simulink model "IndustrialMicrogrid"  (R2025a)
settings: Solver=FixedStepAuto  StartTime=0.0  StopTime=8  FixedStep=Ts  RelTol=1e-3
PostLoadFcn:
  | IndustrialMicrogridInputData
  | GfmGridFormingConverterInputParameters
model workspace (MAT data in the model file):
  caseNum = 2
undefined symbols (not defined in the file): base, BESS, DiscIntNeverNeededParam, grid, Grid, gridInverter, machine, microgrid, PV, PVInverter, PVTransformer, scrFactorRg, scrFactorXg, transformer, Transition_and_Dispatch_ControlModeType, Ts
libraries: ee_lib x126, fl_lib x91, eeGeneralControl x73, nesl_utility x50, nesl_utility_internal x46, simulink x30, eeTransforms x11, eeSinusoidalMeasurementV2 x5, eeTotalHarmonicDistorsion x4, slpidlib x3, simulink_extras x2, eePowerMeasurement x2
(part 7 of 12)

== system IndustrialMicrogrid/MG2 Primary Substation/PCC Measurements and PCC Breaker/Circuit Breaker ==
  BRK : Inport
  Data Type Conversion : DataTypeConversion  OutDataTypeStr=double  SaturateOnIntegerOverflow=off  RndMeth=Floor
  Open Resistance : Gain  Gain=5e6
  Phase Splitter : ee_lib/Connectors & References/Phase Splitter
  Phase Splitter1 : ee_lib/Connectors & References/Phase Splitter
  Simulink-PS Converter : nesl_utility/Simulink-PS Converter  PhysicalDomain=network_engine_domain  SubClassName=ps_input  LeftPortType=input  RightPortType=output  PseudoPeriodic=off  Frequencies=[]  NoiseDistribution=none  NoiseParameters=[]  Unit=1  AffineConversion=off  FilteringAndDerivatives=provide  SimscapeFilterOrder=1  InputFilterTimeConstant=0.001  UdotUserProvided=0
  Variable Resistor : fl_lib/Electrical/Electrical Elements/Variable Resistor  Rmin=1e-3 Ohm  thermalEnable=false  thermal_mass=1 J/K  i_specify=off  i_priority=None  i=0 A  i_nominal_specify=off  i_nominal_value=1  i_nominal_unit=A  v_specify=off  v_priority=None  v=0 V  v_nominal_specify=off  v_nominal_value=1  v_nominal_unit=V  T_specify=off  T_priority=None  T=300 K  T_nominal_specify=off  T_nominal_value=1  T_nominal_unit=K
  Variable Resistor1 : fl_lib/Electrical/Electrical Elements/Variable Resistor  Rmin=1e-3 Ohm  thermalEnable=false  thermal_mass=1 J/K  i_specify=off  i_priority=None  i=0 A  i_nominal_specify=off  i_nominal_value=1  i_nominal_unit=A  v_specify=off  v_priority=None  v=0 V  v_nominal_specify=off  v_nominal_value=1  v_nominal_unit=V  T_specify=off  T_priority=None  T=300 K  T_nominal_specify=off  T_nominal_value=1  T_nominal_unit=K
  Variable Resistor2 : fl_lib/Electrical/Electrical Elements/Variable Resistor  Rmin=1e-3 Ohm  thermalEnable=false  thermal_mass=1 J/K  i_specify=off  i_priority=None  i=0 A  i_nominal_specify=off  i_nominal_value=1  i_nominal_unit=A  v_specify=off  v_priority=None  v=0 V  v_nominal_specify=off  v_nominal_value=1  v_nominal_unit=V  T_specify=off  T_priority=None  T=300 K  T_nominal_specify=off  T_nominal_value=1  T_nominal_unit=K
  In : PMIOPort  Side=Left
  ~ : PMIOPort  Port=2  Side=Right
  wires:
  Data Type Conversion/1 -> Open Resistance/1
  BRK/1 -> Data Type Conversion/1
  Open Resistance/1 -> Simulink-PS Converter/1
  connections:
  Phase Splitter1/RConn2 -- Variable Resistor1/RConn1
  Variable Resistor1/LConn2 -- Phase Splitter/RConn2
  Phase Splitter1/RConn3 -- Variable Resistor2/RConn1
  Phase Splitter/RConn1 -- Variable Resistor/LConn2
  Variable Resistor2/LConn2 -- Phase Splitter/RConn3
  Phase Splitter1/RConn1 -- Variable Resistor/RConn1
  Phase Splitter1/LConn1 -- ~/RConn1
  Variable Resistor/LConn1 -- Simulink-PS Converter/RConn1 -- Variable Resistor2/LConn1 -- Variable Resistor1/LConn1
  Phase Splitter/LConn1 -- In/RConn1

== system IndustrialMicrogrid/MG2 Primary Substation/PCC Measurements and PCC Breaker/Grid Current Measurement ==
  Current and Voltage Sensor (Three-Phase)1 : ee_lib/Sensors & Transducers/Current and Voltage Sensor (Three-Phase)  vMeasurementType=ee.enum.vmeasurement.ll  outputUnit=ee.enum.unit.pu  SRated=2.5e6 A*V  VRated=microgrid.voltage V  I_specify=off  I_priority=None  I=[0, 0, 0] A  I_nominal_specify=off  I_nominal_value=1  I_nominal_unit=A  V_specify=off  V_priority=None  V=[0, 0, 0] V  V_nominal_specify=off  V_nominal_value=1  V_nominal_unit=V
      settings: InternalSimscapePortConfiguration="{\"Bottom\":[],\"Left\":[{\"id\":\"N1\",\"label\":\"~1\",\"type\":\"foundation.electrical.three_phase\"}],\"Right\":[{\"id\":\"V_output\",\"label\":\"V\",\"type\":\"output\"},{\"id\":\"I_output\",\"label\":\"I\",\"type\":\"output\"},{\"id\":\"N2\",\"label\":\"~2\",\"type\":\"foundation.electrical.three_phase\"}],\"Top\":[]}"
  PS-Simulink Converter2 : nesl_utility_internal/PS-Simulink Converter  PhysicalDomain=network_engine_domain  SubClassName=ps_output  LeftPortType=input  RightPortType=output  PseudoPeriodic=off  Frequencies=[]  VectorFormat=1-D array  Unit=V  AffineConversion=off
  PS-Simulink Converter3 : nesl_utility_internal/PS-Simulink Converter  PhysicalDomain=network_engine_domain  SubClassName=ps_output  LeftPortType=input  RightPortType=output  PseudoPeriodic=off  Frequencies=[]  VectorFormat=1-D array  Unit=A  AffineConversion=off
  Terminator : Terminator
  ~ : PMIOPort  Side=Left
  "~ " : PMIOPort  Port=2  Side=Right
  Out Bus Element : Outport  PortName=Grid  Element=voltage
  wires:
  PS-Simulink Converter3/1 -> Terminator/1
  PS-Simulink Converter2/1 -> Out Bus Element/1
  connections:
  Current and Voltage Sensor (Three-Phase)1/RConn3 -- "~ "/RConn1
  Current and Voltage Sensor (Three-Phase)1/RConn2 -- PS-Simulink Converter3/LConn1
  ~/RConn1 -- Current and Voltage Sensor (Three-Phase)1/LConn1
  Current and Voltage Sensor (Three-Phase)1/RConn1 -- PS-Simulink Converter2/LConn1

== system IndustrialMicrogrid/MG2 Primary Substation/PCC Measurements and PCC Breaker/Grid Power Measurement ==
  Current and Voltage Sensor (Three-Phase) : ee_lib/Sensors & Transducers/Current and Voltage Sensor (Three-Phase)  vMeasurementType=ee.enum.vmeasurement.ll  outputUnit=ee.enum.unit.pu  SRated=2.5e6 A*V  VRated=microgrid.voltage V  I_specify=off  I_priority=None  I=[0, 0, 0] A  I_nominal_specify=off  I_nominal_value=1  I_nominal_unit=A  V_specify=off  V_priority=None  V=[0, 0, 0] V  V_nominal_specify=off  V_nominal_value=1  V_nominal_unit=V
      settings: InternalSimscapePortConfiguration="{\"Bottom\":[],\"Left\":[{\"id\":\"N1\",\"label\":\"~1\",\"type\":\"foundation.electrical.three_phase\"}],\"Right\":[{\"id\":\"V_output\",\"label\":\"V\",\"type\":\"output\"},{\"id\":\"I_output\",\"label\":\"I\",\"type\":\"output\"},{\"id\":\"N2\",\"label\":\"~2\",\"type\":\"foundation.electrical.three_phase\"}],\"Top\":[]}"
  Low-Pass Filter (Discrete or Continuous) : eeGeneralControl/Low-Pass Filter (Discrete or Continuous)  K=1  T=0.1  B=inf  A=-inf  init_option=Inherited from block input  x0=0  Ts=Ts
  Low-Pass Filter (Discrete or Continuous)1 : eeGeneralControl/Low-Pass Filter (Discrete or Continuous)  K=1  T=0.1  B=inf  A=-inf  init_option=Inherited from block input  x0=0  Ts=Ts
  PS-Simulink Converter : nesl_utility_internal/PS-Simulink Converter  PhysicalDomain=network_engine_domain  SubClassName=ps_output  LeftPortType=input  RightPortType=output  PseudoPeriodic=off  Frequencies=[]  VectorFormat=1-D array  Unit=inherit  AffineConversion=off
  PS-Simulink Converter1 : nesl_utility_internal/PS-Simulink Converter  PhysicalDomain=network_engine_domain  SubClassName=ps_output  LeftPortType=input  RightPortType=output  PseudoPeriodic=off  Frequencies=[]  VectorFormat=1-D array  Unit=inherit  AffineConversion=off
  PS-Simulink Converter8 : nesl_utility_internal/PS-Simulink Converter  PhysicalDomain=network_engine_domain  SubClassName=ps_output  LeftPortType=input  RightPortType=output  PseudoPeriodic=off  Frequencies=[]  VectorFormat=1-D array  Unit=MW  AffineConversion=off
  PS-Simulink Converter9 : nesl_utility_internal/PS-Simulink Converter  PhysicalDomain=network_engine_domain  SubClassName=ps_output  LeftPortType=input  RightPortType=output  PseudoPeriodic=off  Frequencies=[]  VectorFormat=1-D array  Unit=MV*A  AffineConversion=off
  Power Sensor (Three-Phase)2 : ee_lib/Sensors & Transducers/Power Sensor (Three-Phase)  load_type=ee.enum.passive.type_balanced.balanced  f0=60 Hz  config=ee.enum.with_neutral.no  rho=1
      settings: InternalSimscapePortConfiguration="{\"Bottom\":[],\"Left\":[{\"id\":\"N1\",\"label\":\"~1\",\"type\":\"foundation.electrical.three_phase\"}],\"Right\":[{\"id\":\"N2\",\"label\":\"~2\",\"type\":\"foundation.electrical.three_phase\"}],\"Top\":[{\"id\":\"Pm\",\"label\":\"P\",\"type\":\"output\"},{\"id\":\"Qm\",\"label\":\"Q\",\"type\":\"output\"}]}"
  ~ : PMIOPort  Side=Left
  "~ " : PMIOPort  Port=2  Side=Right
  Out Bus Element : Outport  PortName=PCC  Element=voltage
  Out Bus Element1 : Outport  PortName=PCC  Element=current
  Out Bus Element2 : Outport  PortName=PCC  Element=activePower
  Out Bus Element3 : Outport  PortName=PCC  Element=reactivePower
  wires:
  Low-Pass Filter (Discrete or Continuous)1/1 -> Out Bus Element3/1
  Low-Pass Filter (Discrete or Continuous)/1 -> Out Bus Element2/1
  PS-Simulink Converter1/1 -> Out Bus Element1/1
  PS-Simulink Converter/1 -> Out Bus Element/1
  PS-Simulink Converter9/1 -> Low-Pass Filter (Discrete or Continuous)1/1
  PS-Simulink Converter8/1 -> Low-Pass Filter (Discrete or Continuous)/1
  connections:
  ~/RConn1 -- Power Sensor (Three-Phase)2/LConn1
  PS-Simulink Converter8/LConn1 -- Power Sensor (Three-Phase)2/LConn2
  Current and Voltage Sensor (Three-Phase)/RConn3 -- "~ "/RConn1
  PS-Simulink Converter9/LConn1 -- Power Sensor (Three-Phase)2/LConn3
  Power Sensor (Three-Phase)2/RConn1 -- Current and Voltage Sensor (Three-Phase)/LConn1
  PS-Simulink Converter/LConn1 -- Current and Voltage Sensor (Three-Phase)/RConn1
  Current and Voltage Sensor (Three-Phase)/RConn2 -- PS-Simulink Converter1/LConn1

== system IndustrialMicrogrid/MG2 Processing, Lighting and Auxiliary Loads/Motor Loads/Subsystem ==
  Gain : Gain  Commented=on  Gain=60/(2*pi)
  Ideal Rotational Motion Sensor : fl_lib/Mechanical/Mechanical Sensors/Ideal Rotational Motion Sensor  Commented=on  reference=foundation.enum.MeasurementReference.difference  acceleration_port=false  velocity_port=true  position_port=false  wrap_angle=false  offset=0 rad
      settings: InternalSimscapePortConfiguration="{\"Bottom\":[],\"Left\":[{\"id\":\"R\",\"label\":\"R\",\"type\":\"foundation.mechanical.rotational.rotational\"}],\"Right\":[{\"id\":\"C\",\"label\":\"C\",\"type\":\"foundation.mechanical.rotational.rotational\"},{\"id\":\"W\",\"label\":\"W\",\"type\":\"output\"}],\"Top\":[]}"
  Machine Mechanical Power : ee_lib/Electromechanical/Mechanical/Machine Mechanical Power  power_sign=1  SRated=750000 A*V  FRated=60 Hz  nPolePairs=2  inputUnit=ee.enum.unit.si  torque_factor=2  inertia_option=2  J=10 kg*m^2  H=3.525 W*s/(A*V)  damper_option=2  D=39.0509 N*m*s/rad  pu_D=0.01  initialization_option=1  fMechanical0=30 Hz  fElectrical0=0 Hz
      settings: InternalSimscapePortConfiguration="{\"Bottom\":[],\"Left\":[{\"id\":\"Pm\",\"label\":\"Pm\",\"type\":\"input\"}],\"Right\":[{\"id\":\"R\",\"label\":\"R\",\"type\":\"foundation.mechanical.rotational.rotational\"},{\"id\":\"C\",\"label\":\"C\",\"type\":\"foundation.mechanical.rotational.rotational\"}],\"Top\":[]}"
  Mechanical Rotational Reference : fl_lib/Mechanical/Rotational Elements/Mechanical Rotational Reference
  PS Constant : fl_lib/Physical Signals/Sources/PS Constant  Commented=on  constant=300000
  PS Step : fl_lib/Physical Signals/Sources/PS Step  step_time=1e-3 s  initial_value=0  final_value=300000
  PS-Simulink Converter : nesl_utility/PS-Simulink Converter  Commented=on  PhysicalDomain=network_engine_domain  SubClassName=ps_output  LeftPortType=input  RightPortType=output  PseudoPeriodic=off  Frequencies=[]  VectorFormat=inherit  Unit=inherit  AffineConversion=off
  Rotational Friction : fl_lib/Mechanical/Rotational Elements/Rotational Friction  brkwy_trq=25 N*m  brkwy_vel=0.1 rad/s  Col_trq=20 N*m  visc_coef=0.001 N*m*s/rad  w_specify=on  w_priority=None  w=0 rad/s  w_nominal_specify=off  w_nominal_value=1  w_nominal_unit=rad/s  t_specify=on  t_priority=None  t=0 N*m  t_nominal_specify=off  t_nominal_value=1  t_nominal_unit=N*m
  Scope : Scope  Commented=on
      settings: ActiveDisplayYMinimum=566.67789  ActiveDisplayYMaximum=1937.03579
  Step : Step  Commented=on  Time=0.05  After=300000  SampleTime=0
  Conn1 : PMIOPort  Side=Left
  Conn2 : PMIOPort  Port=2  Side=Left
  wires:
  Gain/1 -> Scope/1
  PS-Simulink Converter/1 -> Gain/1
  connections:
  Ideal Rotational Motion Sensor/RConn1 -- Machine Mechanical Power/RConn2 -- Rotational Friction/RConn1 -- Conn2/RConn1 -- Mechanical Rotational Reference/LConn1
  Machine Mechanical Power/RConn1 -- Rotational Friction/LConn1 -- Conn1/RConn1 -- Ideal Rotational Motion Sensor/LConn1
  PS-Simulink Converter/LConn1 -- Ideal Rotational Motion Sensor/RConn2
  PS Step/RConn1 -- Machine Mechanical Power/LConn1

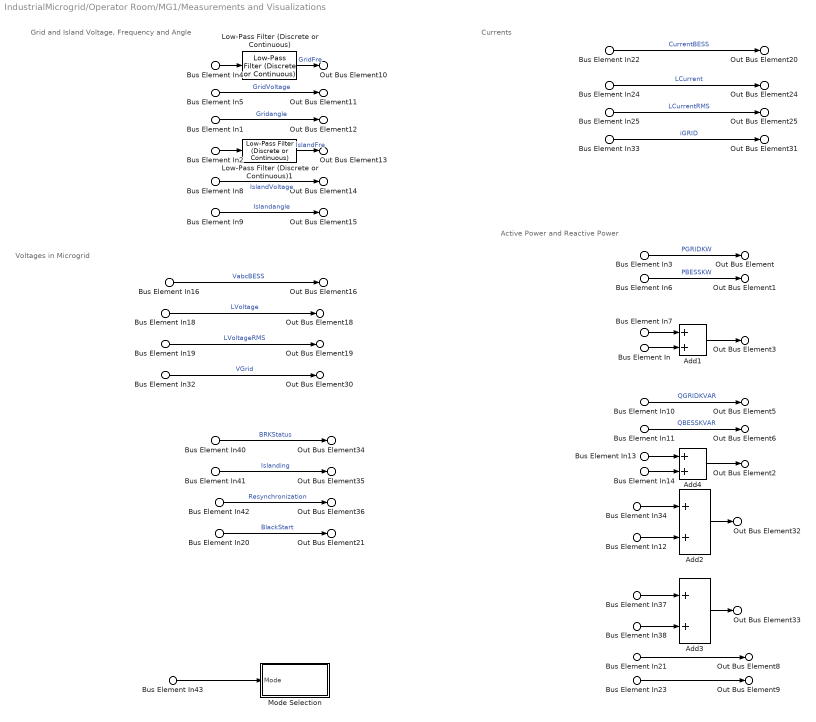
== system IndustrialMicrogrid/Operator Room/MG1/Measurements and Visualizations  ==
  note: Currents
  note: Voltages in Microgrid
  note: Grid and Island Voltage, Frequency and Angle
  note: Active Power and Reactive Power
  Bus Element In4 : Inport  PortName=MG1  Element=MGController.mPLL.Grid.frequency
  Bus Element In5 : Inport  PortName=MG1  Element=MGController.mPLL.Grid.voltage
  Bus Element In1 : Inport  PortName=MG1  Element=MGController.mPLL.Grid.angle
  Bus Element In2 : Inport  PortName=MG1  Element=MGController.mPLL.Island.frequency
  Bus Element In8 : Inport  PortName=MG1  Element=MGController.mPLL.Island.voltage
  Bus Element In9 : Inport  PortName=MG1  Element=MGController.mPLL.Island.angle
  Bus Element In40 : Inport  PortName=MG1  Element=MGController.BRK Status
  Bus Element In41 : Inport  PortName=MG1  Element=MGController.Status.plannedIslandingEnable
  Bus Element In42 : Inport  PortName=MG1  Element=MGController.Status.resyncEnable
  Bus Element In43 : Inport  PortName=MG1  Element=MGController.Status.mode
  Bus Element In20 : Inport  PortName=MG1  Element=MGController.Status.blackStartEnable
  Bus Element In10 : Inport  PortName=MG1  Element=mPCC.PCC.reactivePower
  Bus Element In37 : Inport  PortName=MG1  Element=mPCC.PCC.reactivePower
  Bus Element In32 : Inport  PortName=MG1  Element=mPCC.PCC.voltage
  Bus Element In33 : Inport  PortName=MG1  Element=mPCC.PCC.current
  Bus Element In3 : Inport  PortName=MG1  Element=mPCC.PCC.activePower
  Bus Element In34 : Inport  PortName=MG1  Element=mPCC.PCC.activePower
  Bus Element In6 : Inport  PortName=MG1  Element=mBESS.active power
  Bus Element In12 : Inport  PortName=MG1  Element=mBESS.active power
  Bus Element In11 : Inport  PortName=MG1  Element=mBESS.reactive power
  Bus Element In38 : Inport  PortName=MG1  Element=mBESS.reactive power
  Bus Element In16 : Inport  PortName=MG1  Element=mBESS.voltage
  Bus Element In22 : Inport  PortName=MG1  Element=mBESS.current
  Bus Element In7 : Inport  Port=2  PortName=mLoad  Element=activePower
  Bus Element In18 : Inport  Port=2  PortName=mLoad  Element=voltage
  Bus Element In19 : Inport  Port=2  PortName=mLoad  Element=voltageRMS
  Bus Element In24 : Inport  Port=2  PortName=mLoad  Element=current
  Bus Element In25 : Inport  Port=2  PortName=mLoad  Element=currentRMS
  Bus Element In13 : Inport  Port=2  PortName=mLoad  Element=reactivePower
  Bus Element In : Inport  Port=3  PortName=mLoad3  Element=activePower
  Bus Element In14 : Inport  Port=3  PortName=mLoad3  Element=reactivePower
  Bus Element In21 : Inport  Port=4  PortName=mTieline  Element=activePower
  Bus Element In23 : Inport  Port=4  PortName=mTieline  Element=reactivePower
  Add{1..4} (4 alike) : Sum
  Low-Pass Filter (Discrete or Continuous) : eeGeneralControl/Low-Pass Filter (Discrete or Continuous)  K=1  T=0.001  B=inf  A=-inf  init_option=Inherited from block input  x0=0  Ts=-1
  Low-Pass Filter (Discrete or Continuous)1 : eeGeneralControl/Low-Pass Filter (Discrete or Continuous)  K=1  T=0.001  B=inf  A=-inf  init_option=Specify as parameter  x0=0  Ts=-1
  Mode Selection : Subsystem
  Out Bus Element12 : Outport  PortName=Visualization  Element=MG1.Grid.angle
  Out Bus Element : Outport  PortName=Visualization  Element=MG1.Grid.activePower
  Out Bus Element5 : Outport  PortName=Visualization  Element=MG1.Grid.reactivePower
  Out Bus Element10 : Outport  PortName=Visualization  Element=MG1.Grid.frequency
  Out Bus Element11 : Outport  PortName=Visualization  Element=MG1.Grid.voltage
  Out Bus Element13 : Outport  PortName=Visualization  Element=MG1.Island.frequency
  Out Bus Element14 : Outport  PortName=Visualization  Element=MG1.Island.voltage
  Out Bus Element15 : Outport  PortName=Visualization  Element=MG1.Island.angle
  Out Bus Element16 : Outport  PortName=Visualization  Element=MG1.BESS.voltage
  Out Bus Element20 : Outport  PortName=Visualization  Element=MG1.BESS.current
  Out Bus Element1 : Outport  PortName=Visualization  Element=MG1.BESS.activePower
  Out Bus Element6 : Outport  PortName=Visualization  Element=MG1.BESS.reactivePower
  Out Bus Element18 : Outport  PortName=Visualization  Element=MG1.Load.voltage
  Out Bus Element19 : Outport  PortName=Visualization  Element=MG1.Load.voltageRMS
  Out Bus Element25 : Outport  PortName=Visualization  Element=MG1.Load.currentRMS
  Out Bus Element24 : Outport  PortName=Visualization  Element=MG1.Load.current
  Out Bus Element3 : Outport  PortName=Visualization  Element=MG1.Load.activePower
  Out Bus Element2 : Outport  PortName=Visualization  Element=MG1.Load.reactivePower
  Out Bus Element30 : Outport  PortName=Visualization  Element=MG1.PCC.voltage
  Out Bus Element34 : Outport  PortName=Visualization  Element=MG1.PCC.BRKStatus
  Out Bus Element31 : Outport  PortName=Visualization  Element=MG1.PCC.current
  Out Bus Element35 : Outport  PortName=Visualization  Element=MG1.plannedIslanding
  Out Bus Element36 : Outport  PortName=Visualization  Element=MG1.resynchronization
  Out Bus Element21 : Outport  PortName=Visualization  Element=MG1.blackStart
  Out Bus Element32 : Outport  PortName=Visualization  Element=MG1.Generation.activePower
  Out Bus Element33 : Outport  PortName=Visualization  Element=MG1.Generation.reactivePower
  Out Bus Element8 : Outport  PortName=Visualization  Element=MG1.Tieline.activePower
  Out Bus Element9 : Outport  PortName=Visualization  Element=MG1.Tieline.reactivePower
  wires:
  Bus Element In4/1 -> Low-Pass Filter (Discrete or Continuous)/1
  Bus Element In1/1 -> Out Bus Element12/1  "Gridangle"
  Bus Element In9/1 -> Out Bus Element15/1  "Islandangle"
  Bus Element In3/1 -> Out Bus Element/1  "PGRIDKW"
  Bus Element In6/1 -> Out Bus Element1/1  "PBESSKW"
  Bus Element In10/1 -> Out Bus Element5/1  "QGRIDKVAR"
  Bus Element In11/1 -> Out Bus Element6/1  "QBESSKVAR"
  Bus Element In5/1 -> Out Bus Element11/1  "GridVoltage"
  Bus Element In2/1 -> Low-Pass Filter (Discrete or Continuous)1/1
  Bus Element In8/1 -> Out Bus Element14/1  "IslandVoltage"
  Bus Element In16/1 -> Out Bus Element16/1  "VabcBESS"
  Bus Element In18/1 -> Out Bus Element18/1  "LVoltage"
  Bus Element In19/1 -> Out Bus Element19/1  "LVoltageRMS"
  Bus Element In24/1 -> Out Bus Element24/1  "LCurrent"
  Bus Element In22/1 -> Out Bus Element20/1  "CurrentBESS"
  Bus Element In25/1 -> Out Bus Element25/1  "LCurrentRMS"
  Bus Element In32/1 -> Out Bus Element30/1  "VGrid"
  Bus Element In33/1 -> Out Bus Element31/1  "iGRID"
  Bus Element In34/1 -> Add2/1
  Bus Element In38/1 -> Add3/2
  Bus Element In37/1 -> Add3/1
  Add2/1 -> Out Bus Element32/1
  Add3/1 -> Out Bus Element33/1
  Bus Element In40/1 -> Out Bus Element34/1  "BRKStatus"
  Bus Element In41/1 -> Out Bus Element35/1  "Islanding"
  Bus Element In42/1 -> Out Bus Element36/1  "Resynchronization"
  Bus Element In43/1 -> Mode Selection/1(Mode)
  Low-Pass Filter (Discrete or Continuous)/1 -> Out Bus Element10/1  "GridFre"
  Low-Pass Filter (Discrete or Continuous)1/1 -> Out Bus Element13/1  "IslandFre"
  Bus Element In20/1 -> Out Bus Element21/1  "BlackStart"
  Bus Element In12/1 -> Add2/2
  Bus Element In/1 -> Add1/2
  Bus Element In7/1 -> Add1/1
  Add1/1 -> Out Bus Element3/1
  Bus Element In13/1 -> Add4/1
  Add4/1 -> Out Bus Element2/1
  Bus Element In14/1 -> Add4/2
  Bus Element In21/1 -> Out Bus Element8/1
  Bus Element In23/1 -> Out Bus Element9/1

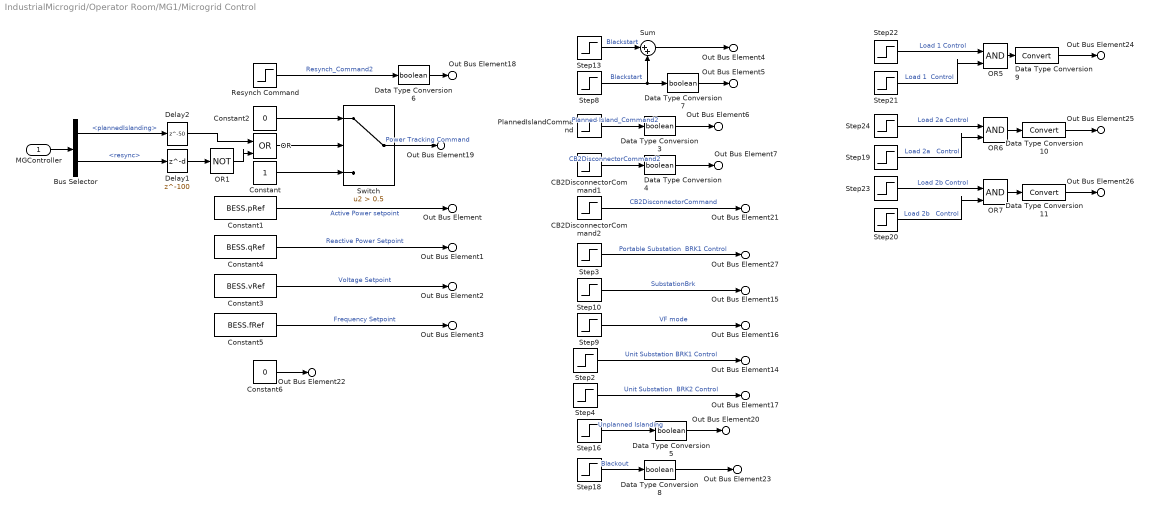
== system IndustrialMicrogrid/Operator Room/MG1/Microgrid Control ==
  MGController : Inport
  Bus Selector : BusSelector  OutputSignals=MGController.Status.plannedIslanding,MGController.Status.resync
  CB2DisconnectorCommand1 : Step  Time=microgrid.controller1PCCBrk  SampleTime=Ts
  CB2DisconnectorCommand2 : Step  Time=microgrid.controller1PCCBrk  SampleTime=Ts
  Constant : Constant
  Constant1 : Constant  Value=BESS.pRef  SampleTime=-1
  Constant2 : Constant  Value=0
  Constant3 : Constant  Value=BESS.vRef  SampleTime=-1
  Constant4 : Constant  Value=BESS.qRef  SampleTime=-1
  Constant5 : Constant  Value=BESS.fRef  SampleTime=-1
  Constant6 : Constant  Value=0
  Data Type Conversion10 : DataTypeConversion  SaturateOnIntegerOverflow=off  RndMeth=Floor
  Data Type Conversion11 : DataTypeConversion  SaturateOnIntegerOverflow=off  RndMeth=Floor
  Data Type Conversion{3..8} (6 alike) : DataTypeConversion  OutDataTypeStr=boolean  SaturateOnIntegerOverflow=off  RndMeth=Floor
  Data Type Conversion9 : DataTypeConversion  SaturateOnIntegerOverflow=off  RndMeth=Floor
  Delay1 : Delay  DelayLength=100  InitialCondition=0  SampleTime=Ts*45*100
  Delay2 : Delay  DelayLength=50  InitialCondition=0  SampleTime=Ts*45
  OR : Logic  Operator=OR  IconShape=distinctive  AllPortsSameDT=off  OutDataTypeStr=boolean
  OR1 : Logic  Operator=NOT  IconShape=distinctive  AllPortsSameDT=off  OutDataTypeStr=boolean
  OR5 : Logic  IconShape=distinctive  AllPortsSameDT=off  OutDataTypeStr=boolean
  OR6 : Logic  IconShape=distinctive  AllPortsSameDT=off  OutDataTypeStr=boolean
  OR7 : Logic  IconShape=distinctive  AllPortsSameDT=off  OutDataTypeStr=boolean
  PlannedIslandCommand : Step  Time=microgrid.controller1PlannedIsland  SampleTime=Ts
  Resynch Command : Step  Time=microgrid.controller1Resynch  SampleTime=Ts
  Step10 : Step  Time=microgrid.controller1SubstationBrk  SampleTime=Ts
  Step13 : Step  Time=microgrid.controller1BlackStart+microgrid.controller1BlackStartDelay  After=-1  SampleTime=Ts
  Step16 : Step  Time=100  SampleTime=Ts
  Step18 : Step  Time=microgrid.controller1Blackout  SampleTime=Ts
  Step19 : Step  Time=microgrid.controller1BlackStart+microgrid.controller1BlackStartDelay+microgrid.controller1BlackStartBlockLoad1PickUp1+microgrid.controller1BlackStartBlockLoad1PickUp2  Before=1  After=0  SampleTime=Ts
  Step2 : Step  Time=microgrid.controller1UnitSubstationBrk1  SampleTime=Ts
  Step20 : Step  Time=microgrid.controller1BlackStart+microgrid.controller1BlackStartDelay+microgrid.controller2BlackStartBlockLoad1PickUp1+microgrid.controller1BlackStartBlockLoad1PickUp2+microgrid.controller1BlackStartBlockLoad1PickUp3  Before=1  SampleTime=Ts
  Step21 : Step  Time=microgrid.controller1BlackStart+microgrid.controller1BlackStartDelay+microgrid.controller1BlackStartBlockLoad1PickUp1  Before=1  After=0  SampleTime=Ts
  Step22 : Step  Time=microgrid.controller1Load1Control  Before=1  After=0  SampleTime=Ts
  Step23 : Step  Time=microgrid.controller1Load2Control  Before=1  After=0  SampleTime=Ts
  Step24 : Step  Time=microgrid.controller1Load2Control  Before=1  After=0  SampleTime=Ts
  Step3 : Step  Time=microgrid.controller1PortableSubstationBrk  Before=1  After=0  SampleTime=Ts
  Step4 : Step  Time=microgrid.controller1UnitSubstationBrk2  SampleTime=Ts
  Step8 : Step  Time=microgrid.controller1BlackStart  SampleTime=Ts
  Step9 : Step  Time=microgrid.controller1VFMode  SampleTime=Ts
  Sum : Sum  Inputs=|++
  Switch : Switch  Criteria=u2 > Threshold  Threshold=0.5  SaturateOnIntegerOverflow=off  InputSameDT=off
  Out Bus Element : Outport  PortName=CtrlRm  Element=MG1.BESS.PRef
  Out Bus Element1 : Outport  PortName=CtrlRm  Element=MG1.BESS.QRef
  Out Bus Element2 : Outport  PortName=CtrlRm  Element=MG1.BESS.VRef
  Out Bus Element3 : Outport  PortName=CtrlRm  Element=MG1.BESS.FRef
  Out Bus Element22 : Outport  PortName=CtrlRm  Element=MG1.BESSReactivePower
  Out Bus Element4 : Outport  PortName=CtrlRm  Element=MG1.blackStartReset
  Out Bus Element5 : Outport  PortName=CtrlRm  Element=MG1.blackStart
  Out Bus Element6 : Outport  PortName=CtrlRm  Element=MG1.plannedIslanding
  Out Bus Element7 : Outport  PortName=CtrlRm  Element=MG1.plannedIslanding1
  Out Bus Element18 : Outport  PortName=CtrlRm  Element=MG1.Resync
  Out Bus Element19 : Outport  PortName=CtrlRm  Element=MG1.PowerCmd
  Out Bus Element21 : Outport  PortName=CtrlRm  Element=MG1.BRKcontrol
  Out Bus Element15 : Outport  PortName=CtrlRm  Element=MG1.Substation.brk
  Out Bus Element16 : Outport  PortName=CtrlRm  Element=MG1.VFMode
  Out Bus Element27 : Outport  PortName=CtrlRm  Element=MG1.PortableSubstationBrk1
  Out Bus Element20 : Outport  PortName=CtrlRm  Element=MG1.unplannedIslanding
  Out Bus Element23 : Outport  PortName=CtrlRm  Element=MG1.blackout
  Out Bus Element14 : Outport  PortName=CtrlRm  Element=MG1.UnitSubstation.Brk1
  Out Bus Element17 : Outport  PortName=CtrlRm  Element=MG1.UnitSubstation.Brk2
  Out Bus Element24 : Outport  PortName=CtrlRm  Element=MG1.Load.Load1Control
  Out Bus Element25 : Outport  PortName=CtrlRm  Element=MG1.Load.Load2aControl
  Out Bus Element26 : Outport  PortName=CtrlRm  Element=MG1.Load.Load2bControl
  wires:
  OR/1 -> Switch/2
  Constant/1 -> Switch/3
  CB2DisconnectorCommand1/1 -> Data Type Conversion4/1  "CB2DisconnectorCommand2"
  Switch/1 -> Out Bus Element19/1  "Power Tracking Command"
  Resynch Command/1 -> Data Type Conversion6/1  "Resynch_Command2"
  Delay2/1 -> OR/1
  Constant3/1 -> Out Bus Element2/1  "Voltage Setpoint"
  Constant5/1 -> Out Bus Element3/1  "Frequency Setpoint"
  PlannedIslandCommand/1 -> Data Type Conversion3/1  "Planned Island_Command2"
  Bus Selector/1 -> Delay2/1  "<plannedIslanding>"
  Sum/1 -> Out Bus Element4/1
  Step8/1 -> Data Type Conversion7/1, Sum/2  "Blackstart"
  Constant4/1 -> Out Bus Element1/1  "Reactive Power Setpoint"
  Constant2/1 -> Switch/1
  Delay1/1 -> OR1/1
  MGController/1 -> Bus Selector/1
  Step13/1 -> Sum/1  "Blackstart"
  Constant1/1 -> Out Bus Element/1  "Active Power setpoint"
  OR1/1 -> OR/2
  Bus Selector/2 -> Delay1/1  "<resync>"
  Step16/1 -> Data Type Conversion5/1  "Unplanned Islanding"
  Constant6/1 -> Out Bus Element22/1
  Data Type Conversion3/1 -> Out Bus Element6/1
  Data Type Conversion4/1 -> Out Bus Element7/1
  Data Type Conversion5/1 -> Out Bus Element20/1
  Data Type Conversion6/1 -> Out Bus Element18/1
  Data Type Conversion7/1 -> Out Bus Element5/1
  Step18/1 -> Data Type Conversion8/1  "Blackout"
  Data Type Conversion8/1 -> Out Bus Element23/1
  OR5/1 -> Data Type Conversion9/1
  Step20/1 -> OR7/2  "Load 2b   Control"
  Step19/1 -> OR6/2  "Load 2a   Control"
  Step22/1 -> OR5/1  "Load 1 Control"
  Data Type Conversion9/1 -> Out Bus Element24/1
  Data Type Conversion11/1 -> Out Bus Element26/1
  OR7/1 -> Data Type Conversion11/1
  Data Type Conversion10/1 -> Out Bus Element25/1
  OR6/1 -> Data Type Conversion10/1
  Step21/1 -> OR5/2  "Load 1  Control"
  Step24/1 -> OR6/1  "Load 2a Control"
  Step23/1 -> OR7/1  "Load 2b Control"
  Step10/1 -> Out Bus Element15/1  "SubstationBrk"
  Step4/1 -> Out Bus Element17/1  "Unit Substation  BRK2 Control"
  Step2/1 -> Out Bus Element14/1  "Unit Substation BRK1 Control"
  Step3/1 -> Out Bus Element27/1  "Portable Substation  BRK1 Control"
  Step9/1 -> Out Bus Element16/1  "VF mode"
  CB2DisconnectorCommand2/1 -> Out Bus Element21/1  "CB2DisconnectorCommand"

== system IndustrialMicrogrid/Operator Room/MG1/Monitoring of system performance ==
  Bus Element In : Inport  PortName=Visualization  Element=MG1.Load.voltage
  BusElementIn6 : Inport  PortName=Visualization  Element=MG1.Load.activePower
  BusElementIn7 : Inport  PortName=Visualization  Element=MG1.Load.reactivePower
  BusElementIn1 : Inport  PortName=Visualization  Element=MG1.Island.frequency
  BusElementIn2 : Inport  PortName=Visualization  Element=MG1.Island.voltage
  BusElementIn5 : Inport  PortName=Visualization  Element=MG1.Generation.activePower
  BusElementIn8 : Inport  PortName=Visualization  Element=MG1.Generation.reactivePower
  BusElementIn4 : Inport  PortName=Visualization  Element=MG1.Tieline.reactivePower
  BusElementIn3 : Inport  PortName=Visualization  Element=MG1.Tieline.activePower
  BusElementIn : Inport  PortName=Visualization  Element=MG1.BESS.voltage
  Add : Sum  Inputs=++-
  Add1 : Sum  Inputs=++-
  Low-Pass Filter (Discrete or Continuous)1 : eeGeneralControl/Low-Pass Filter (Discrete or Continuous)  K=1  T=0.04  B=inf  A=-inf  init_option=Specify as parameter  x0=0  Ts=-1
  Terminator{,1..5} (6 alike) : Terminator
  Total Harmonic Distortion : eeTotalHarmonicDistorsion/Total Harmonic Distortion  f=60  Ts=-1
  Total Harmonic Distortion2 : eeTotalHarmonicDistorsion/Total Harmonic Distortion  f=60  Ts=-1
  wires:
  Bus Element In/1 -> Total Harmonic Distortion/1
  Total Harmonic Distortion/1 -> Terminator/1  "Load Voltage THD (%)"
  BusElementIn/1 -> Total Harmonic Distortion2/1
  Total Harmonic Distortion2/1 -> Terminator1/1  "PCC Voltage THD (%)"
  BusElementIn3/1 -> Add/2
  BusElementIn5/1 -> Add/1
  BusElementIn6/1 -> Add/3
  Add/1 -> Terminator2/1
  BusElementIn8/1 -> Add1/1
  BusElementIn4/1 -> Add1/2
  BusElementIn7/1 -> Add1/3
  Add1/1 -> Terminator3/1
  BusElementIn1/1 -> Low-Pass Filter (Discrete or Continuous)1/1
  Low-Pass Filter (Discrete or Continuous)1/1 -> Terminator4/1  "IslandFre"
  BusElementIn2/1 -> Terminator5/1

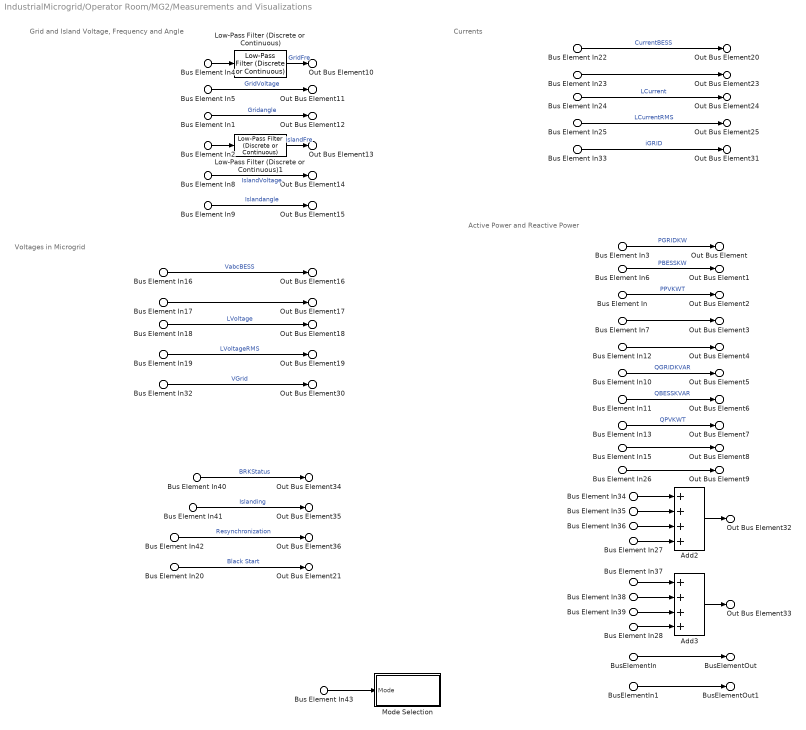
== system IndustrialMicrogrid/Operator Room/MG2/Measurements and Visualizations ==
  note: Currents
  note: Voltages in Microgrid
  note: Grid and Island Voltage, Frequency and Angle
  note: Active Power and Reactive Power
  Bus Element In4 : Inport  PortName=MG2  Element=MGController.mPLL.Grid.frequency
  Bus Element In5 : Inport  PortName=MG2  Element=MGController.mPLL.Grid.voltage
  Bus Element In1 : Inport  PortName=MG2  Element=MGController.mPLL.Grid.angle
  Bus Element In2 : Inport  PortName=MG2  Element=MGController.mPLL.Island.frequency
  Bus Element In8 : Inport  PortName=MG2  Element=MGController.mPLL.Island.voltage
  Bus Element In9 : Inport  PortName=MG2  Element=MGController.mPLL.Island.angle
  Bus Element In40 : Inport  PortName=MG2  Element=MGController.BRK Status
  Bus Element In41 : Inport  PortName=MG2  Element=MGController.Status.plannedIslandingEnable
  Bus Element In43 : Inport  PortName=MG2  Element=MGController.Status.mode
  Bus Element In20 : Inport  PortName=MG2  Element=MGController.Status.blackStartEnable
  Bus Element In42 : Inport  PortName=MG2  Element=MGController.Status.resyncEnable
  Bus Element In10 : Inport  PortName=MG2  Element=mPCC.PCC.reactivePower
  Bus Element In37 : Inport  PortName=MG2  Element=mPCC.PCC.reactivePower
  Bus Element In32 : Inport  PortName=MG2  Element=mPCC.PCC.voltage
  Bus Element In33 : Inport  PortName=MG2  Element=mPCC.PCC.current
  Bus Element In3 : Inport  PortName=MG2  Element=mPCC.PCC.activePower
  Bus Element In34 : Inport  PortName=MG2  Element=mPCC.PCC.activePower
  Bus Element In6 : Inport  PortName=MG2  Element=mBESS.active power
  Bus Element In35 : Inport  PortName=MG2  Element=mBESS.active power
  Bus Element In11 : Inport  PortName=MG2  Element=mBESS.reactive power
  Bus Element In38 : Inport  PortName=MG2  Element=mBESS.reactive power
  Bus Element In16 : Inport  PortName=MG2  Element=mBESS.voltage
  Bus Element In22 : Inport  PortName=MG2  Element=mBESS.current
  Bus Element In17 : Inport  Port=2  PortName=mPV  Element=PV.voltage
  Bus Element In13 : Inport  Port=2  PortName=mPV  Element=PV.rectivePower
  Bus Element In39 : Inport  Port=2  PortName=mPV  Element=PV.rectivePower
  Bus Element In36 : Inport  Port=2  PortName=mPV  Element=PV.activePower
  Bus Element In : Inport  Port=2  PortName=mPV  Element=PV.activePower
  Bus Element In23 : Inport  Port=2  PortName=mPV  Element=PV.current
  Bus Element In7 : Inport  Port=3  PortName=mLoad2  Element=active power
  Bus Element In15 : Inport  Port=3  PortName=mLoad2  Element=reactive power
  Bus Element In18 : Inport  Port=3  PortName=mLoad2  Element=voltage
  Bus Element In19 : Inport  Port=3  PortName=mLoad2  Element=voltageRMS
  Bus Element In24 : Inport  Port=3  PortName=mLoad2  Element=current
  Bus Element In25 : Inport  Port=3  PortName=mLoad2  Element=currentRMS
  Bus Element In12 : Inport  Port=4  PortName=mPowerCentre  Element=diesel.active power
  Bus Element In27 : Inport  Port=4  PortName=mPowerCentre  Element=diesel.active power
  Bus Element In26 : Inport  Port=4  PortName=mPowerCentre  Element=diesel.reactive power
  Bus Element In28 : Inport  Port=4  PortName=mPowerCentre  Element=diesel.reactive power
  BusElementIn : Inport  Port=4  PortName=mPowerCentre  Element=tieline.activepower
  BusElementIn1 : Inport  Port=4  PortName=mPowerCentre  Element=tieline.reactivepower
  Add2 : Sum  Inputs=++++
  Add3 : Sum  Inputs=++++
  Low-Pass Filter (Discrete or Continuous) : eeGeneralControl/Low-Pass Filter (Discrete or Continuous)  K=1  T=0.001  B=inf  A=-inf  init_option=Inherited from block input  x0=0  Ts=-1
  Low-Pass Filter (Discrete or Continuous)1 : eeGeneralControl/Low-Pass Filter (Discrete or Continuous)  K=1  T=0.001  B=inf  A=-inf  init_option=Specify as parameter  x0=0  Ts=-1
  Mode Selection : Subsystem
  Out Bus Element10 : Outport  PortName=Visualization  Element=MG2.Grid.frequency
  Out Bus Element11 : Outport  PortName=Visualization  Element=MG2.Grid.voltage
  Out Bus Element12 : Outport  PortName=Visualization  Element=MG2.Grid.angle
  Out Bus Element : Outport  PortName=Visualization  Element=MG2.Grid.activePower
  Out Bus Element5 : Outport  PortName=Visualization  Element=MG2.Grid.reactivePower
  Out Bus Element13 : Outport  PortName=Visualization  Element=MG2.Island.frequency
  Out Bus Element14 : Outport  PortName=Visualization  Element=MG2.Island.voltage
  Out Bus Element15 : Outport  PortName=Visualization  Element=MG2.Island.angle
  Out Bus Element16 : Outport  PortName=Visualization  Element=MG2.BESS.voltage
  Out Bus Element20 : Outport  PortName=Visualization  Element=MG2.BESS.current
  Out Bus Element1 : Outport  PortName=Visualization  Element=MG2.BESS.activePower
  Out Bus Element6 : Outport  PortName=Visualization  Element=MG2.BESS.reactivePower
  Out Bus Element17 : Outport  PortName=Visualization  Element=MG2.PV.ACVoltage
  Out Bus Element23 : Outport  PortName=Visualization  Element=MG2.PV.ACCurrent
  Out Bus Element2 : Outport  PortName=Visualization  Element=MG2.PV.activePower
  Out Bus Element7 : Outport  PortName=Visualization  Element=MG2.PV.reactivePower
  Out Bus Element18 : Outport  PortName=Visualization  Element=MG2.Load.voltage
  Out Bus Element19 : Outport  PortName=Visualization  Element=MG2.Load.voltageRMS
  Out Bus Element25 : Outport  PortName=Visualization  Element=MG2.Load.currentRMS
  Out Bus Element24 : Outport  PortName=Visualization  Element=MG2.Load.current
  Out Bus Element3 : Outport  PortName=Visualization  Element=MG2.Load.activePower
  Out Bus Element8 : Outport  PortName=Visualization  Element=MG2.Load.reactivePower
  Out Bus Element30 : Outport  PortName=Visualization  Element=MG2.PCC.voltage
  Out Bus Element34 : Outport  PortName=Visualization  Element=MG2.PCC.BRKStatus
  Out Bus Element31 : Outport  PortName=Visualization  Element=MG2.PCC.current
  Out Bus Element35 : Outport  PortName=Visualization  Element=MG2.plannedIslanding
  Out Bus Element36 : Outport  PortName=Visualization  Element=MG2.resynchronization
  Out Bus Element21 : Outport  PortName=Visualization  Element=MG2.blackStart
  Out Bus Element32 : Outport  PortName=Visualization  Element=MG2.Generation.activePower
  Out Bus Element33 : Outport  PortName=Visualization  Element=MG2.Generation.reactivePower
  Out Bus Element4 : Outport  PortName=Visualization  Element=MG2.Diesel.activePower
  Out Bus Element9 : Outport  PortName=Visualization  Element=MG2.Diesel.reactivePower
  BusElementOut : Outport  PortName=Visualization  Element=Tieline.activepower
  BusElementOut1 : Outport  PortName=Visualization  Element=Tieline.reactivepower
  wires:
  Bus Element In4/1 -> Low-Pass Filter (Discrete or Continuous)/1
  Bus Element In1/1 -> Out Bus Element12/1  "Gridangle"
  Bus Element In9/1 -> Out Bus Element15/1  "Islandangle"
  Bus Element In3/1 -> Out Bus Element/1  "PGRIDKW"
  Bus Element In6/1 -> Out Bus Element1/1  "PBESSKW"
  Bus Element In/1 -> Out Bus Element2/1  "PPVKWT"
  Bus Element In7/1 -> Out Bus Element3/1
  Bus Element In10/1 -> Out Bus Element5/1  "QGRIDKVAR"
  Bus Element In11/1 -> Out Bus Element6/1  "QBESSKVAR"
  Bus Element In13/1 -> Out Bus Element7/1  "QPVKWT"
  Bus Element In15/1 -> Out Bus Element8/1
  Bus Element In5/1 -> Out Bus Element11/1  "GridVoltage"
  Bus Element In2/1 -> Low-Pass Filter (Discrete or Continuous)1/1
  Bus Element In8/1 -> Out Bus Element14/1  "IslandVoltage"
  Bus Element In16/1 -> Out Bus Element16/1  "VabcBESS"
  Bus Element In17/1 -> Out Bus Element17/1
  Bus Element In18/1 -> Out Bus Element18/1  "LVoltage"
  Bus Element In19/1 -> Out Bus Element19/1  "LVoltageRMS"
  Bus Element In23/1 -> Out Bus Element23/1
  Bus Element In24/1 -> Out Bus Element24/1  "LCurrent"
  Bus Element In22/1 -> Out Bus Element20/1  "CurrentBESS"
  Bus Element In25/1 -> Out Bus Element25/1  "LCurrentRMS"
  Bus Element In32/1 -> Out Bus Element30/1  "VGrid"
  Bus Element In33/1 -> Out Bus Element31/1  "iGRID"
  Bus Element In34/1 -> Add2/1
  Bus Element In35/1 -> Add2/2
  Bus Element In36/1 -> Add2/3
  Bus Element In38/1 -> Add3/2
  Bus Element In39/1 -> Add3/3
  Bus Element In37/1 -> Add3/1
  Add2/1 -> Out Bus Element32/1
  Add3/1 -> Out Bus Element33/1
  Bus Element In40/1 -> Out Bus Element34/1  "BRKStatus"
  Bus Element In41/1 -> Out Bus Element35/1  "Islanding"
  Bus Element In42/1 -> Out Bus Element36/1  "Resynchronization"
  Bus Element In43/1 -> Mode Selection/1(Mode)
  Low-Pass Filter (Discrete or Continuous)/1 -> Out Bus Element10/1  "GridFre"
  Low-Pass Filter (Discrete or Continuous)1/1 -> Out Bus Element13/1  "IslandFre"
  Bus Element In20/1 -> Out Bus Element21/1  "Black Start"
  Bus Element In12/1 -> Out Bus Element4/1
  Bus Element In26/1 -> Out Bus Element9/1
  Bus Element In27/1 -> Add2/4
  Bus Element In28/1 -> Add3/4
  BusElementIn/1 -> BusElementOut/1
  BusElementIn1/1 -> BusElementOut1/1

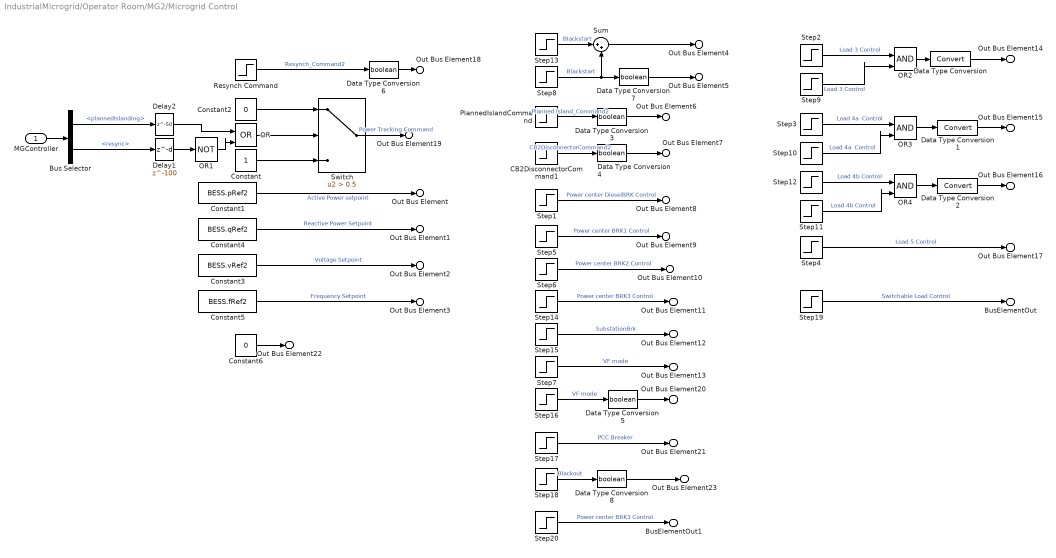
== system IndustrialMicrogrid/Operator Room/MG2/Microgrid Control ==
  MGController : Inport
  Bus Selector : BusSelector  OutputSignals=MGController.Status.plannedIslanding,MGController.Status.resync
  CB2DisconnectorCommand1 : Step  Time=microgrid.controller2PCCBrk  SampleTime=Ts
  Constant : Constant
  Constant1 : Constant  Value=BESS.pRef2  SampleTime=-1
  Constant2 : Constant  Value=0
  Constant3 : Constant  Value=BESS.vRef2  SampleTime=-1
  Constant4 : Constant  Value=BESS.qRef2  SampleTime=-1
  Constant5 : Constant  Value=BESS.fRef2  SampleTime=-1
  Constant6 : Constant  Value=0
  Data Type Conversion : DataTypeConversion  SaturateOnIntegerOverflow=off  RndMeth=Floor
  Data Type Conversion1 : DataTypeConversion  SaturateOnIntegerOverflow=off  RndMeth=Floor
  Data Type Conversion2 : DataTypeConversion  SaturateOnIntegerOverflow=off  RndMeth=Floor
  Data Type Conversion{3..8} (6 alike) : DataTypeConversion  OutDataTypeStr=boolean  SaturateOnIntegerOverflow=off  RndMeth=Floor
  Delay1 : Delay  DelayLength=100  InitialCondition=0  SampleTime=Ts*45
  Delay2 : Delay  DelayLength=50  InitialCondition=0  SampleTime=Ts*45
  OR : Logic  Operator=OR  IconShape=distinctive  AllPortsSameDT=off  OutDataTypeStr=boolean
  OR1 : Logic  Operator=NOT  IconShape=distinctive  AllPortsSameDT=off  OutDataTypeStr=boolean
  OR2 : Logic  IconShape=distinctive  AllPortsSameDT=off  OutDataTypeStr=boolean
  OR3 : Logic  IconShape=distinctive  AllPortsSameDT=off  OutDataTypeStr=boolean
  OR4 : Logic  IconShape=distinctive  AllPortsSameDT=off  OutDataTypeStr=boolean
  PlannedIslandCommand : Step  Time=microgrid.controller2PlannedIsland  SampleTime=Ts
  Resynch Command : Step  Time=microgrid.controller2Resynch  SampleTime=Ts
  Step1 : Step  Time=microgrid.controller2DieselBrk  SampleTime=Ts
  Step10 : Step  Time=microgrid.controller2BlackStart+microgrid.controller2BlackStartDelay+microgrid.controller2BlackStartBlockLoad1PickUp1+microgrid.controller2BlackStartBlockLoad1PickUp2  Before=1  After=0  SampleTime=Ts
  Step11 : Step  Time=microgrid.controller2BlackStart+microgrid.controller2BlackStartDelay+microgrid.controller2BlackStartBlockLoad1PickUp1+microgrid.controller2BlackStartBlockLoad1PickUp2+microgrid.controller2BlackStartBlockLoad1PickUp3  Before=1  After=0  SampleTime=Ts
  Step12 : Step  Time=microgrid.controller2Load4Control  Before=1  After=0  SampleTime=Ts
  Step13 : Step  Time=microgrid.controller2BlackStart+microgrid.controller2BlackStartDelay  After=-1  SampleTime=Ts
  Step14 : Step  Time=microgrid.controller2PowerCenterBrk3  SampleTime=Ts
  Step15 : Step  Time=microgrid.controller2SubstationBrk  SampleTime=Ts
  Step16 : Step  Time=microgrid.controller2UnplannedIslanding  SampleTime=Ts
  Step17 : Step  Time=100  SampleTime=Ts
  Step18 : Step  Time=microgrid.controller2Blackout  SampleTime=Ts
  Step19 : Step  Time=microgrid.controller2SwitchableLoad  SampleTime=Ts
  Step2 : Step  Time=microgrid.controller2Load3Control  Before=1  After=0  SampleTime=Ts
  Step20 : Step  Time=20  Before=1  After=0  SampleTime=Ts
  Step3 : Step  Time=microgrid.controller2Load4Control  Before=1  After=0  SampleTime=Ts
  Step4 : Step  Time=microgrid.controller2Load5Control  Before=1  After=0  SampleTime=Ts
  Step5 : Step  Time=microgrid.controller2PowerCenterBrk1  Before=1  After=0  SampleTime=Ts
  Step6 : Step  Time=microgrid.controller2PowerCenterBrk2  SampleTime=Ts
  Step7 : Step  Time=microgrid.controller2VFMode  SampleTime=Ts
  Step8 : Step  Time=microgrid.controller2BlackStart  SampleTime=Ts
  Step9 : Step  Time=microgrid.controller2BlackStart+microgrid.controller2BlackStartDelay+microgrid.controller2BlackStartBlockLoad1PickUp1  Before=1  After=0  SampleTime=Ts
  Sum : Sum  Inputs=|++
  Switch : Switch  Criteria=u2 > Threshold  Threshold=0.5  SaturateOnIntegerOverflow=off  InputSameDT=off
  Out Bus Element : Outport  PortName=CtrlRm  Element=MG2.BESS.PRef
  Out Bus Element1 : Outport  PortName=CtrlRm  Element=MG2.BESS.QRef
  Out Bus Element2 : Outport  PortName=CtrlRm  Element=MG2.BESS.VRef
  Out Bus Element3 : Outport  PortName=CtrlRm  Element=MG2.BESS.FRef
  BusElementOut1 : Outport  PortName=CtrlRm  Element=MG2.BESS.CapacitorBRK
  Out Bus Element4 : Outport  PortName=CtrlRm  Element=MG2.blackStartReset
  Out Bus Element5 : Outport  PortName=CtrlRm  Element=MG2.blackStart
  Out Bus Element6 : Outport  PortName=CtrlRm  Element=MG2.plannedIslanding
  Out Bus Element7 : Outport  PortName=CtrlRm  Element=MG2.plannedIslanding1
  Out Bus Element8 : Outport  PortName=CtrlRm  Element=MG2.PowerCentre.dieselBrk
  Out Bus Element9 : Outport  PortName=CtrlRm  Element=MG2.PowerCentre.brk1
  Out Bus Element10 : Outport  PortName=CtrlRm  Element=MG2.PowerCentre.brk2
  Out Bus Element11 : Outport  PortName=CtrlRm  Element=MG2.PowerCentre.brk3
  BusElementOut : Outport  PortName=CtrlRm  Element=MG2.PowerCentre.brk4
  Out Bus Element12 : Outport  PortName=CtrlRm  Element=MG2.Substation.brk
  Out Bus Element13 : Outport  PortName=CtrlRm  Element=MG2.VFMode
  Out Bus Element18 : Outport  PortName=CtrlRm  Element=MG2.Resync
  Out Bus Element19 : Outport  PortName=CtrlRm  Element=MG2.PowerCmd
  Out Bus Element14 : Outport  PortName=CtrlRm  Element=MG2.Load.Load3
  Out Bus Element15 : Outport  PortName=CtrlRm  Element=MG2.Load.Load4a
  Out Bus Element16 : Outport  PortName=CtrlRm  Element=MG2.Load.Load4b
  Out Bus Element17 : Outport  PortName=CtrlRm  Element=MG2.Load.Load5
  Out Bus Element20 : Outport  PortName=CtrlRm  Element=MG2.unplannedIslanding
  Out Bus Element21 : Outport  PortName=CtrlRm  Element=MG2.BRKcontrol
  Out Bus Element22 : Outport  PortName=CtrlRm  Element=MG2.BESSReactivePower
  Out Bus Element23 : Outport  PortName=CtrlRm  Element=MG2.blackout
  wires:
  Step11/1 -> OR4/2  "Load 4b Control"
  Step10/1 -> OR3/2  "Load 4a  Control"
  Step15/1 -> Out Bus Element12/1  "SubstationBrk"
  Step9/1 -> OR2/2  "Load 3 Control"
  OR3/1 -> Data Type Conversion1/1
  Step12/1 -> OR4/1  "Load 4b Control"
  Step1/1 -> Out Bus Element8/1  "Power center DieselBRK Control"
  OR/1 -> Switch/2
  Constant/1 -> Switch/3
  CB2DisconnectorCommand1/1 -> Data Type Conversion4/1  "CB2DisconnectorCommand2"
  Step6/1 -> Out Bus Element10/1  "Power center BRK2 Control"
  Data Type Conversion/1 -> Out Bus Element14/1
  Switch/1 -> Out Bus Element19/1  "Power Tracking Command"
  OR2/1 -> Data Type Conversion/1
  Step3/1 -> OR3/1  "Load 4a  Control"
  Step4/1 -> Out Bus Element17/1  "Load 5 Control"
  Step2/1 -> OR2/1  "Load 3 Control"
  OR4/1 -> Data Type Conversion2/1
  Data Type Conversion2/1 -> Out Bus Element16/1
  Resynch Command/1 -> Data Type Conversion6/1  "Resynch_Command2"
  Delay2/1 -> OR/1
  Step7/1 -> Out Bus Element13/1  "VF mode"
  Step5/1 -> Out Bus Element9/1  "Power center BRK1 Control"
  Data Type Conversion1/1 -> Out Bus Element15/1
  Constant3/1 -> Out Bus Element2/1  "Voltage Setpoint"
  Constant5/1 -> Out Bus Element3/1  "Frequency Setpoint"
  PlannedIslandCommand/1 -> Data Type Conversion3/1  "Planned Island_Command2"
  Bus Selector/1 -> Delay2/1  "<plannedIslanding>"
  Sum/1 -> Out Bus Element4/1
  Step8/1 -> Data Type Conversion7/1, Sum/2  "Blackstart"
  Step14/1 -> Out Bus Element11/1  "Power center BRK3 Control"
  Constant4/1 -> Out Bus Element1/1  "Reactive Power Setpoint"
  Constant2/1 -> Switch/1
  Delay1/1 -> OR1/1
  MGController/1 -> Bus Selector/1
  Step13/1 -> Sum/1  "Blackstart"
  Constant1/1 -> Out Bus Element/1  "Active Power setpoint"
  OR1/1 -> OR/2
  Bus Selector/2 -> Delay1/1  "<resync>"
  Step16/1 -> Data Type Conversion5/1  "VF mode"
  Step17/1 -> Out Bus Element21/1  "PCC Breaker"
  Constant6/1 -> Out Bus Element22/1
  Data Type Conversion3/1 -> Out Bus Element6/1
  Data Type Conversion4/1 -> Out Bus Element7/1
  Data Type Conversion5/1 -> Out Bus Element20/1
  Data Type Conversion6/1 -> Out Bus Element18/1
  Data Type Conversion7/1 -> Out Bus Element5/1
  Step18/1 -> Data Type Conversion8/1  "Blackout"
  Data Type Conversion8/1 -> Out Bus Element23/1
  Step19/1 -> BusElementOut/1  "Switchable Load Control"
  Step20/1 -> BusElementOut1/1  "Power center BRK3 Control"

== system IndustrialMicrogrid/Operator Room/MG2/Monitoring of system performance ==
  Bus Element In : Inport  PortName=Visualization  Element=MG2.Load.voltage
  BusElementIn6 : Inport  PortName=Visualization  Element=MG2.Load.activePower
  BusElementIn7 : Inport  PortName=Visualization  Element=MG2.Load.reactivePower
  BusElementIn : Inport  PortName=Visualization  Element=MG2.PCC.voltage
  BusElementIn1 : Inport  PortName=Visualization  Element=MG2.Island.frequency
  BusElementIn2 : Inport  PortName=Visualization  Element=MG2.Island.voltage
  BusElementIn5 : Inport  PortName=Visualization  Element=MG2.Generation.activePower
  BusElementIn8 : Inport  PortName=Visualization  Element=MG2.Generation.reactivePower
  BusElementIn3 : Inport  PortName=Visualization  Element=Tieline.activepower
  BusElementIn4 : Inport  PortName=Visualization  Element=Tieline.reactivepower
  Add : Sum  Inputs=++-
  Add1 : Sum  Inputs=++-
  Low-Pass Filter (Discrete or Continuous)1 : eeGeneralControl/Low-Pass Filter (Discrete or Continuous)  K=1  T=0.04  B=inf  A=-inf  init_option=Specify as parameter  x0=0  Ts=-1
  Terminator{,1..5} (6 alike) : Terminator
  Total Harmonic Distortion : eeTotalHarmonicDistorsion/Total Harmonic Distortion  f=60  Ts=-1
  Total Harmonic Distortion2 : eeTotalHarmonicDistorsion/Total Harmonic Distortion  f=60  Ts=-1
  wires:
  Total Harmonic Distortion/1 -> Terminator/1  "Load Voltage THD (%)"
  Total Harmonic Distortion2/1 -> Terminator1/1  "PCC Voltage THD (%)"
  BusElementIn3/1 -> Add/2
  BusElementIn5/1 -> Add/1
  BusElementIn6/1 -> Add/3
  Add/1 -> Terminator2/1
  BusElementIn8/1 -> Add1/1
  BusElementIn4/1 -> Add1/2
  BusElementIn7/1 -> Add1/3
  Add1/1 -> Terminator3/1
  BusElementIn1/1 -> Low-Pass Filter (Discrete or Continuous)1/1
  BusElementIn2/1 -> Terminator5/1
  Low-Pass Filter (Discrete or Continuous)1/1 -> Terminator4/1  "IslandFre"
  Bus Element In/1 -> Total Harmonic Distortion/1
  BusElementIn/1 -> Total Harmonic Distortion2/1
